simulink model "statefdbk_real"  (R2015a)
settings: Solver=ode3  StartTime=0  StopTime=20  RelTol=1e-3
values from neighbouring files (symbols this model uses):
  A = [A zeros(n,1); -C_ 1]    [control_integral.m]    (also in model.mat = [2.19826062055 1 0 0 0 0 -0.950981109251 0 1 0 0 0 ... (36 e; square_2V_2_5hz_100fs.mat = [3.68944323306 1 0 0 0 0 0 0 0 0 0 -4.87835143564 ... (121 e; square_2V_2_5hz_50fs.mat = [3.32314178319 1 0 0 0 0 0 0 0 0 0 -4.05203564565 ... (121 e)
  B = [B ; 0]    [control_integral.m]    (also in model.mat = [1 0 0 0 0 0]; square_2V_2_5hz_100fs.mat = [1 0 0 0 0 0 0 0 0 0 0]; square_2V_2_5hz_50fs.mat = [1 0 0 0 0 0 0 0 0 0 0])
  C_ = C    [control.m]    (also in control_integral.m)
  K = dlqr(A,B,Q,R)    [control.m]    (also in control_integral.m = K(1:end-1))
  L = dlqe(A,G,C,Q_w,R_v)    [control.m]    (also in control_integral.m; plotter.m = convlength(L,'in','m')*100)
  N = inv(C_*inv(eye(n)-A+B*K)*B)    [control_integral.m]    (also in model_identification_ecpd.m = length(u))
undefined symbols (not defined in the file or in its folder): MIO, National_Instruments, PCI
libraries: sldrtlib x3
settings Model: SimulationMode=external  ExtModeTrigDuration=100001  Creator=Alunos  LastModifiedBy=Alunos
settings DataIOCC: SaveFormat=StructureWithTime
settings HardwareCC: ProdIntDivRoundTo=Zero  ProdEndianess=LittleEndian  ProdHWDeviceType=Intel->x86/Pentium  TargetIntDivRoundTo=Zero  TargetEndianess=LittleEndian  TargetHWDeviceType=Intel->x86/Pentium
settings RTWCC: SystemTargetFile=rtwin.tlc  TemplateMakefile=rtwin.tmf  Description=Simulink Desktop Real-Time  RTWCompilerOptimization=on
settings CodeAppCC: MaxIdLength=95
settings RTWinTargetCC: TargetPreCompLibLocation=C:\Program Files\MATLAB\R2015a\toolbox\sldrt\lib\win32

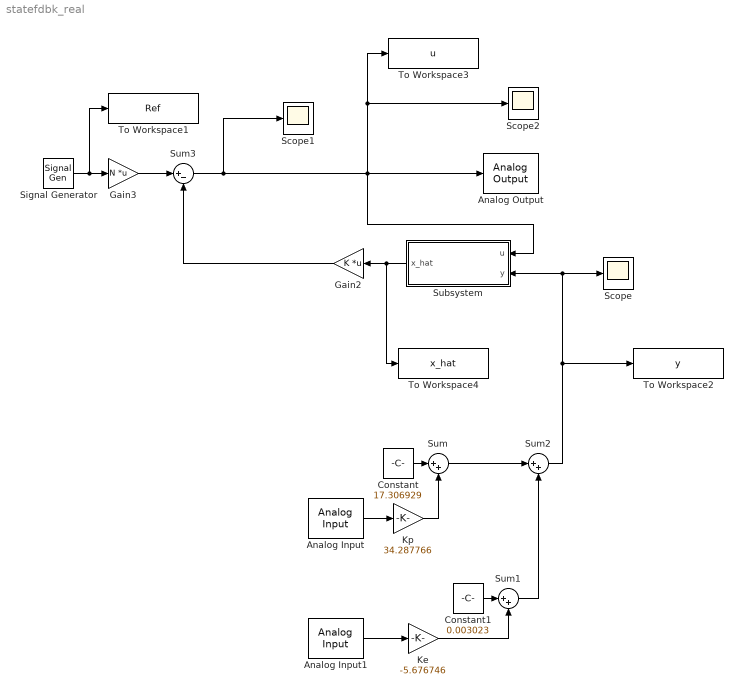
== system statefdbk_real ==
  Analog Input : sldrtlib/Analog Input  SampleTime=0.02  MaxMissedTicks=10  ShowMissedTicks=off  YieldWhenWaiting=off  DrvName=National_Instruments/PCI-MIO-16E-4  DrvAddress=4294967295  DrvOptions=[0 0 0 0 0 0]  Channels=1  RangeMode=1  VoltRange=1  DataType=1
      settings: AttributesFormatString=National Instruments\nPCI-MIO-16E-4 [auto]
  Analog Input1 : sldrtlib/Analog Input  SampleTime=0.02  MaxMissedTicks=10  ShowMissedTicks=off  YieldWhenWaiting=off  DrvName=National_Instruments/PCI-MIO-16E-4  DrvAddress=4294967295  DrvOptions=[0 0 0 0 0 0]  Channels=2  RangeMode=1  VoltRange=1  DataType=1
      settings: AttributesFormatString=National Instruments\nPCI-MIO-16E-4 [auto]
  Analog Output : sldrtlib/Analog Output  SampleTime=0.02  MaxMissedTicks=10  ShowMissedTicks=off  YieldWhenWaiting=off  DrvName=National_Instruments/PCI-MIO-16E-4  DrvAddress=4294967295  DrvOptions=[0 0 0 0 0 0]  Channels=1  RangeMode=1  VoltRange=1  InitialValue=0  FinalValue=0
      settings: AttributesFormatString=National Instruments\nPCI-MIO-16E-4 [auto]
  Constant : Constant  Value=17.306929
  Constant1 : Constant  Value=0.003023
  Gain2 : Gain  Gain=K  Multiplication=Matrix(K*u)
  Gain3 : Gain  Gain=N  Multiplication=Matrix(K*u)
  Ke : Gain  Gain=-5.676746
  Kp : Gain  Gain=34.287766
  Scope : Scope
      settings: YMin=-25  YMax=25
  Scope1 : Scope
      settings: YMin=-4  YMax=4  SaveName=ScopeData2
  Scope2 : Scope
      settings: YMin=-5.57682  YMax=2.90692
  Signal Generator : SignalGenerator  WaveForm=square  Amplitude=20  Frequency=0.25
  Subsystem : Subsystem
  Sum : Sum  Inputs=|++
  Sum1 : Sum  Inputs=|++
  Sum2 : Sum  Inputs=|++
  Sum3 : Sum  Inputs=|+-
  To Workspace1 : ToWorkspace  VariableName=Ref  SampleTime=-1
  To Workspace2 : ToWorkspace  VariableName=y  SampleTime=-1
  To Workspace3 : ToWorkspace  VariableName=u  SampleTime=-1
  To Workspace4 : ToWorkspace  VariableName=x_hat  SampleTime=-1
  wires:
  Analog Input/1 -> Kp/1
  Analog Input1/1 -> Ke/1
  Constant/1 -> Sum/1
  Kp/1 -> Sum/2
  Constant1/1 -> Sum1/1
  Ke/1 -> Sum1/2
  Subsystem/1(x_hat) -> To Workspace4/1, Gain2/1
  Sum1/1 -> Sum2/2
  Sum/1 -> Sum2/1
  Sum2/1 -> To Workspace2/1, Subsystem/2(y), Scope/1
  Gain3/1 -> Sum3/1
  Signal Generator/1 -> To Workspace1/1, Gain3/1
  Gain2/1 -> Sum3/2
  Sum3/1 -> Subsystem/1(u), Analog Output/1, To Workspace3/1, Scope2/1, Scope1/1

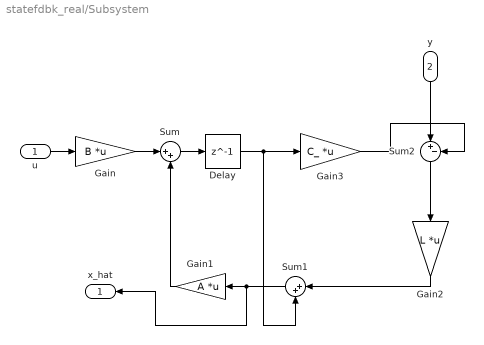
== system statefdbk_real/Subsystem ==
  u : Inport
  y : Inport  Port=2
  Delay : Delay  DelayLength=1  InitialCondition=0
  Gain : Gain  Gain=B  Multiplication=Matrix(K*u)
  Gain1 : Gain  Gain=A  Multiplication=Matrix(K*u)
  Gain2 : Gain  Gain=L  Multiplication=Matrix(K*u)
  Gain3 : Gain  Gain=C_  Multiplication=Matrix(K*u)
  Sum : Sum  Inputs=|++
  Sum1 : Sum  Inputs=|++
  Sum2 : Sum  Inputs=|+-
  x_hat : Outport
  wires:
  u/1 -> Gain/1
  Gain3/1 -> Sum2/2
  y/1 -> Sum2/1
  Sum2/1 -> Gain2/1
  Gain2/1 -> Sum1/1
  Delay/1 -> Sum1/2, Gain3/1
  Sum1/1 -> x_hat/1, Gain1/1
  Gain/1 -> Sum/1
  Sum/1 -> Delay/1
  Gain1/1 -> Sum/2
